simulink model "s4dot2_11leijiaqishinengzixitong"  (R2023b)
settings: Solver=VariableStepAuto  StartTime=0.0  StopTime=10  MaxStep=0.01  RelTol=1e-3
settings Model: Creator=lxj  LastModifiedBy=lxj

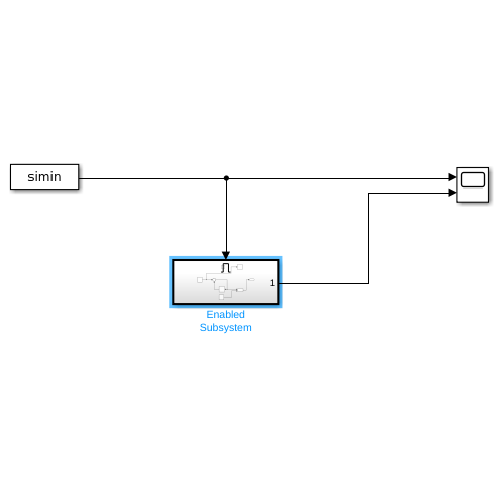
[thumbnail: Simulink's stored preview of the top-level diagram]
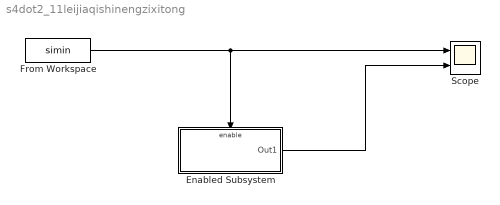
== system s4dot2_11leijiaqishinengzixitong ==
  Enabled Subsystem : Subsystem  TreatAsAtomicUnit=on
  From Workspace : FromWorkspace  VariableName=simin
  Scope : Scope  NumInputPorts=2
  wires:
  From Workspace/1 -> Enabled Subsystem/Enable, Scope/1
  Enabled Subsystem/1(Out1) -> Scope/2

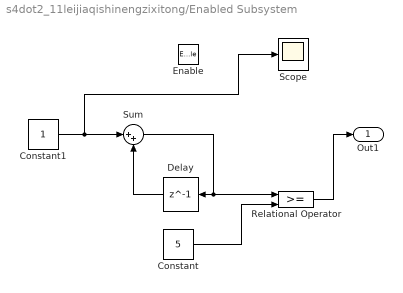
== system s4dot2_11leijiaqishinengzixitong/Enabled Subsystem ==
  Enable : EnablePort  StatesWhenEnabling=reset
  Constant : Constant  Value=5  SampleTime=1
  Constant1 : Constant  SampleTime=1
  Delay : Delay  DelayLength=1  InitialCondition=0  SampleTime=1
  Relational Operator : RelationalOperator  OutDataTypeStr=boolean  RndMeth=Simplest  InputSameDT=off
  Scope : Scope
  Sum : Sum  Inputs=|++
  Out1 : Outport
  wires:
  Constant1/1 -> Scope/1, Sum/1
  Sum/1 -> Relational Operator/1, Delay/1
  Delay/1 -> Sum/2
  Constant/1 -> Relational Operator/2
  Relational Operator/1 -> Out1/1
